simulink model "agingTest"  (R2022a)
settings: configuration reference "agingTestConfig" (kept outside this file)
settings Model: Creator=mateu  LastModifiedBy=mateu
settings ConfigSetRef: SourceName=agingTestConfig  SourceLocation=Base Workspace

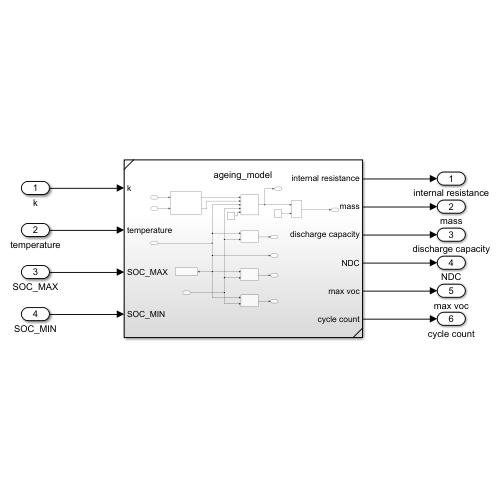
[thumbnail: Simulink's stored preview of the top-level diagram]
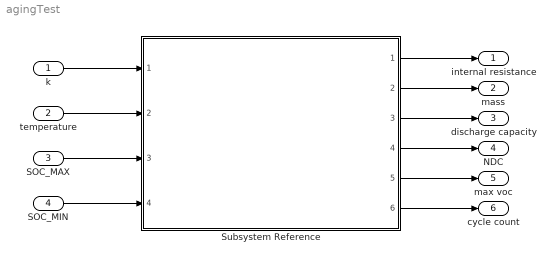
== system agingTest ==
  k : Inport
  temperature : Inport  Port=2
  SOC_MAX : Inport  Port=3
  SOC_MIN : Inport  Port=4
  Subsystem Reference : Subsystem  ReferencedSubsystem=ageing_model
  internal resistance : Outport
  mass : Outport  Port=2
  discharge capacity : Outport  Port=3
  NDC : Outport  Port=4
  max voc : Outport  Port=5
  cycle count : Outport  Port=6
  wires:
  Subsystem Reference/4 -> NDC/1
  Subsystem Reference/5 -> max voc/1
  Subsystem Reference/6 -> cycle count/1
  SOC_MAX/1 -> Subsystem Reference/3
  k/1 -> Subsystem Reference/1
  Subsystem Reference/2 -> mass/1
  temperature/1 -> Subsystem Reference/2
  Subsystem Reference/3 -> discharge capacity/1
  Subsystem Reference/1 -> internal resistance/1
  SOC_MIN/1 -> Subsystem Reference/4
